simulink model "controlador2015"  (R2017b)
settings: Solver=VariableStepAuto  StartTime=0.0  StopTime=N  RelTol=1e-3
values from neighbouring files (symbols this model uses):
  R = 0.01    [init.m]
  x0 = [1;1]    [init.m]
undefined symbols (not defined in the file or in its folder): c, C, gama, phi
libraries: simulink x4, dspsrcs4 x1
settings Model: Creator=Raposo  LastModifiedBy=raposo

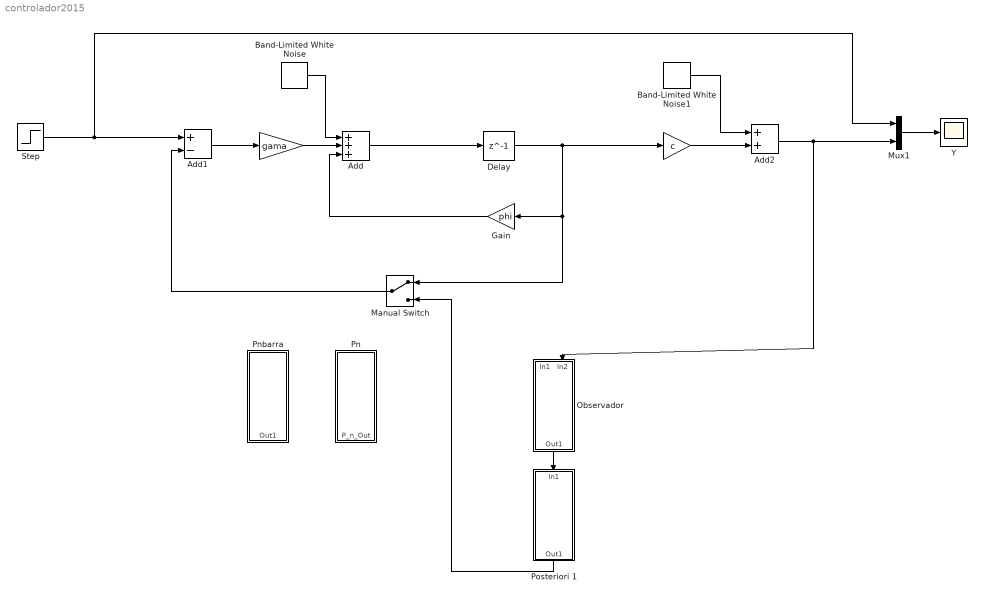
== system controlador2015 ==
  " " : Gain  Gain=c
  " " : Gain  Gain=gama
  " Pn" : Subsystem
  " Pnbarra" : Subsystem
  Add : Sum  Inputs=+++
  Add1 : Sum  Inputs=+-
  Add2 : Sum
  Band-Limited White Noise : simulink/Sources/Band-Limited White Noise  Cov=[0.1]  Ts=0.1  seed=[23341]
  Band-Limited White Noise1 : simulink/Sources/Band-Limited White Noise  Cov=[0.1]  Ts=0.1  seed=[23341]
  Delay : Delay  DelayLength=1  InitialCondition=x0  SampleTime=[1,0]
  Gain : Gain  Gain=phi
  Manual Switch : ManualSwitch
  Mux1 : Mux  Inputs=2
  "Observador " : Subsystem
  Posteriori 1 : Subsystem
  Step : Step  Time=5  SampleTime=0
  Y : Scope
  wires:
  Add/1 -> Delay/1
  Gain/1 -> Add/3
  Delay/1 -> " "/1, Manual Switch/1, Gain/1
  " "/1 -> Add/2
  Add1/1 -> " "/1
  " "/1 -> Add2/2
  Add2/1 -> "Observador "/2(In2), Mux1/2
  Posteriori 1/1(Out1) -> Manual Switch/2
  Mux1/1 -> Y/1
  Step/1 -> Mux1/1, Add1/1
  Band-Limited White Noise/1 -> Add/1
  Band-Limited White Noise1/1 -> Add2/1
  Manual Switch/1 -> Add1/2
  "Observador "/1(Out1) -> Posteriori 1/1(In1)

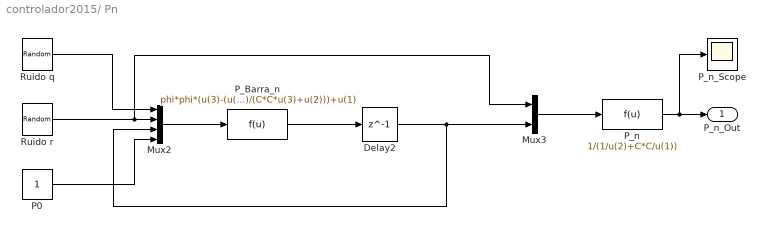
== system controlador2015/ Pn ==
  Delay2 : Delay  DelayLength=1  InitialCondition=0
  Mux2 : Mux
  Mux3 : Mux  Inputs=2
  P0 : Constant  SampleTime=1
  P_Barra_n : Fcn  Expr=phi*phi*(u(3)-(u(3)*u(3)*C*C)/(C*C*u(3)+u(2)))+u(1)
  P_n : Fcn  Expr=1/(1/u(2)+C*C/u(1))
  "P_n_Scope " : Scope
  Ruido q : UniformRandomNumber  SampleTime=0.1
  Ruido r : UniformRandomNumber  SampleTime=0.1
  P_n_Out : Outport
  wires:
  P0/1 -> Mux2/4
  Ruido r/1 -> Mux3/1, Mux2/2
  Ruido q/1 -> Mux2/1
  Delay2/1 -> Mux3/2, Mux2/3
  Mux3/1 -> P_n/1
  P_n/1 -> "P_n_Scope "/1, P_n_Out/1
  Mux2/1 -> P_Barra_n/1
  P_Barra_n/1 -> Delay2/1

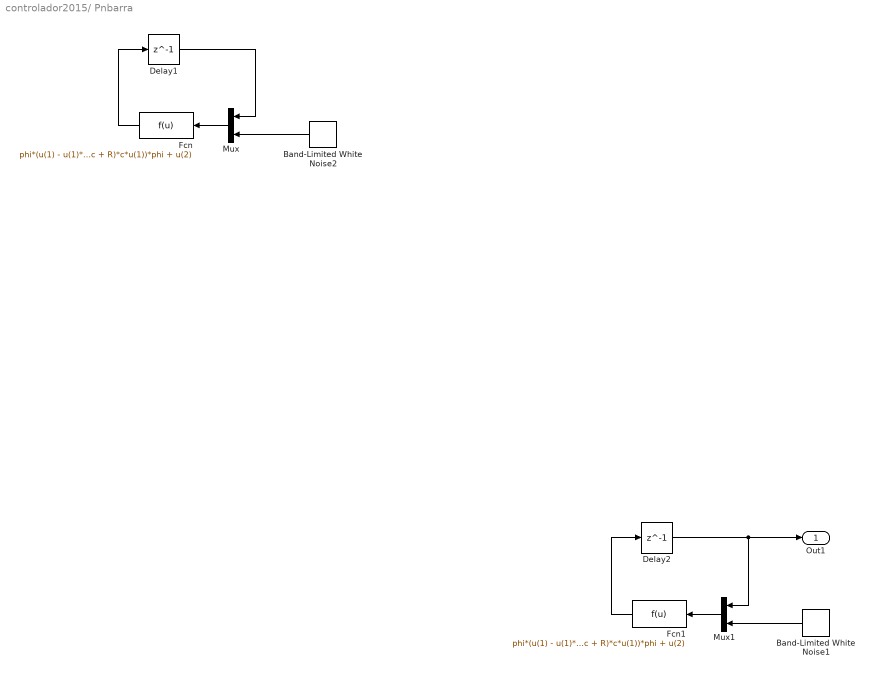
== system controlador2015/ Pnbarra ==
  Band-Limited White Noise1 : simulink/Sources/Band-Limited White Noise  Cov=[0.1]  Ts=0.1  seed=[23341]
  Band-Limited White Noise2 : simulink/Sources/Band-Limited White Noise  Cov=[0.1]  Ts=0.1  seed=[23341]
  Delay1 : Delay  DelayLength=1
  Delay2 : Delay  DelayLength=1
  Fcn : Fcn  Expr=phi*(u(1) - u(1)*c*1/(c*1/u(1)*c + R)*c*u(1))*phi + u(2)
  Fcn1 : Fcn  Expr=phi*(u(1) - u(1)*c*1/(c*1/u(1)*c + R)*c*u(1))*phi + u(2)
  Mux : Mux  Inputs=2
  Mux1 : Mux  Inputs=2
  Out1 : Outport
  wires:
  Mux/1 -> Fcn/1
  Fcn/1 -> Delay1/1
  Band-Limited White Noise2/1 -> Mux/2
  Delay1/1 -> Mux/1
  Mux1/1 -> Fcn1/1
  Fcn1/1 -> Delay2/1
  Band-Limited White Noise1/1 -> Mux1/2
  Delay2/1 -> Out1/1, Mux1/1

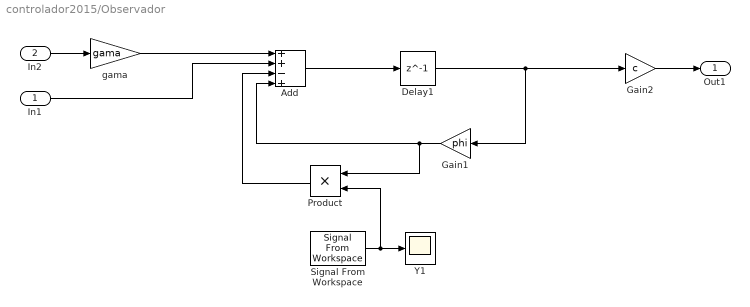
== system controlador2015/Observador  ==
  In1 : Inport
  In2 : Inport  Port=2
  Add : Sum  Inputs=++-+
  Delay1 : Delay  DelayLength=1
  Gain1 : Gain  Gain=phi
  Gain2 : Gain  Gain=c
  Product : Product
  Signal From Workspace : dspsrcs4/Signal From Workspace  X=k  Ts=1  nsamps=1  OutputAfterFinalValue=Setting to zero  ignoreOrWarnInputAndFrameLengths=off  OutputFrames=off
  Y1 : Scope
  "gama " : Gain  Gain=gama
  Out1 : Outport
  wires:
  In1/1 -> Add/2
  Add/1 -> Delay1/1
  Delay1/1 -> Gain2/1, Gain1/1
  Gain1/1 -> Product/1, Add/4
  "gama "/1 -> Add/1
  Gain2/1 -> Out1/1
  In2/1 -> "gama "/1
  Signal From Workspace/1 -> Y1/1, Product/2
  Product/1 -> Add/3

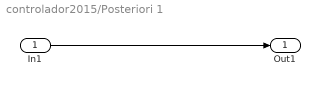
== system controlador2015/Posteriori 1 ==
  In1 : Inport
  Out1 : Outport
  wires:
  In1/1 -> Out1/1
